simulink model "me575_2"  (R2021b)
settings: Solver=VariableStepAuto  StartTime=0.0  StopTime=10.0  RelTol=1e-3
settings Model: Creator=Kumar Chakravarthy  LastModifiedBy=Kumar Chakravarthy

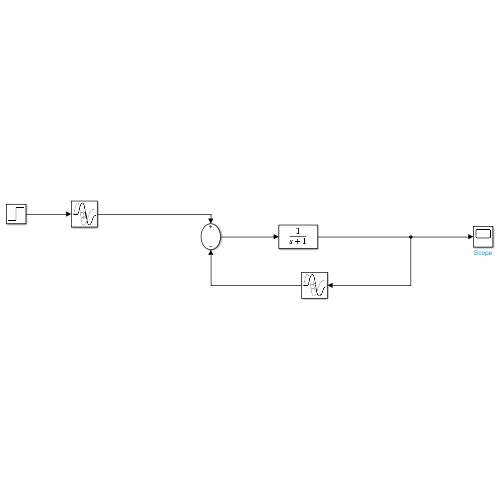
[thumbnail: Simulink's stored preview of the top-level diagram]
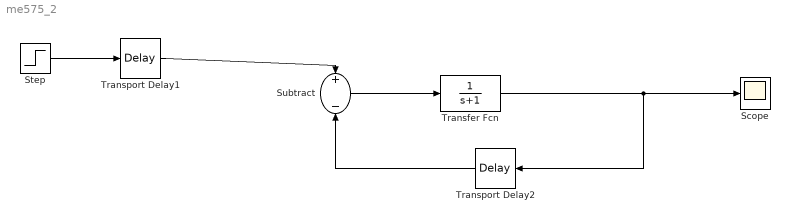
== system me575_2 ==
  Scope : Scope
  Step : Step  SampleTime=0
  Subtract : Sum  Inputs=+-
  Transfer Fcn : TransferFcn  Denominator=[1 1]
  Transport Delay1 : TransportDelay
  Transport Delay2 : TransportDelay
  wires:
  Transfer Fcn/1 -> Transport Delay2/1, Scope/1
  Subtract/1 -> Transfer Fcn/1
  Step/1 -> Transport Delay1/1
  Transport Delay1/1 -> Subtract/1
  Transport Delay2/1 -> Subtract/2
